simulink model "ASM_Traffic_V2X_Complete_Model_2"  (R2019a)
settings: Solver=ode1  StartTime=SIM.tstart.v  StopTime=Inf  FixedStep=SIM.StepSize.v  RelTol=1e-3
PostLoadFcn:
  | if any(exist('dsrtsu_mdlpostloadfcn', 'file') ~= 0), dsrtsu_mdlpostloadfcn('Execute', bdroot); end
  | try, asm_mdl_postloadfcn(bdroot, 'UpdateModel', 2200); catch, disp(lasterr); end,
undefined symbols (not defined in the file): _SensorPnts_1, _SensorPnts_13, _SensorPnts_17, _SensorPnts_21, _SensorPnts_25, _SensorPnts_29, _SensorPnts_33, _SensorPnts_37, _SensorPnts_41, _SensorPnts_45, _SensorPnts_49, _SensorPnts_5, _SensorPnts_53, _SensorPnts_57, _SensorPnts_9, _to_, CPT, G5A, ITS, MDL, rad, s_to_rpm, SIM
libraries: simulink x169, ASM_VehicleDynamics_lib x126, ASM_Traffic_lib x83, ASM_Utils_lib x49, mdbs x45, ASM_Environment_lib x17, dspindex x12, dsaV2xLibraryAux x10, dsmpblib x6, dsaV2xAsn1Library x4, dsaV2xLibrary x4, ASM_BrakeHydraulics_lib x4
(part 30 of 36)

== system ASM_Traffic_V2X_Complete_Model_2/MDLUserInterface/Environment/MDL_DISP/Traffic/Object_Sensor_2D/Object_Sensor_2D_VisualizationData/Sensor_5_Front_Right ==
  Sensor : Inport
  Angle_Hor_Rel[deg] : Gain
  Angle_ScopeZone_Horizontal[deg] : Gain
  Angle_z_Orientation_Sensor_CoorSys_V[deg] : Gain
  Bus Selector : BusSelector  OutputSignals=Parameters.Sensor_Enable[0Off|1On],Parameters.Sensor_Detection_Mode[1Ray|2Sector],Parameters.Length_ScopeZone[m],Parameters.Pos_Sensor_Apex_CoorSys_V[x;y;z][m],Parameters.Angle_z_Orientation_Sensor_CoorSys_V[deg],Parameters.Angle_ScopeZone_Horizontal[deg],Parameters.SensorIdx[],SensorOutput.Object_ID[],SensorOutput.Distance[m],SensorOutput.Angle_Hor_Rel[deg]
  Distance[m] : Gain
  Length_ScopeZone[m] : Gain
  Object_ID[] : Gain
  Pos_Sensor_Apex_CoorSys_V[x;y;z][m] : Gain
  SensorIdx[] : Gain
  Sensor_Detection_Mode[1Ray|2Sector] : Gain
  Sensor_Enable[0Off|1On] : Gain
  Terminator{,1..9} (10 alike) : Terminator
  wires:
  Bus Selector/3 -> Length_ScopeZone[m]/1  "<Length_ScopeZone[m]>"
  Length_ScopeZone[m]/1 -> Terminator9/1
  Bus Selector/10 -> Angle_Hor_Rel[deg]/1  "<Angle_Hor_Rel[deg]>"
  Bus Selector/9 -> Distance[m]/1  "<Distance[m]>"
  Bus Selector/8 -> Object_ID[]/1  "<Object_ID[]>"
  Bus Selector/7 -> SensorIdx[]/1  "<SensorIdx[]>"
  Bus Selector/6 -> Angle_ScopeZone_Horizontal[deg]/1  "<Angle_ScopeZone_Horizontal[deg]>"
  Bus Selector/5 -> Angle_z_Orientation_Sensor_CoorSys_V[deg]/1  "<Angle_z_Orientation_Sensor_CoorSys_V[deg]>"
  Bus Selector/4 -> Pos_Sensor_Apex_CoorSys_V[x;y;z][m]/1  "<Pos_Sensor_Apex_CoorSys_V[x;y;z][m]>"
  Angle_Hor_Rel[deg]/1 -> Terminator8/1
  Distance[m]/1 -> Terminator7/1
  Object_ID[]/1 -> Terminator6/1
  SensorIdx[]/1 -> Terminator5/1
  Angle_ScopeZone_Horizontal[deg]/1 -> Terminator4/1
  Angle_z_Orientation_Sensor_CoorSys_V[deg]/1 -> Terminator3/1
  Pos_Sensor_Apex_CoorSys_V[x;y;z][m]/1 -> Terminator2/1
  Bus Selector/2 -> Sensor_Detection_Mode[1Ray|2Sector]/1  "<Sensor_Detection_Mode[1Ray|2Sector]>"
  Sensor_Detection_Mode[1Ray|2Sector]/1 -> Terminator1/1
  Sensor_Enable[0Off|1On]/1 -> Terminator/1
  Bus Selector/1 -> Sensor_Enable[0Off|1On]/1  "<Sensor_Enable[0Off|1On]>"
  Sensor/1 -> Bus Selector/1

== system ASM_Traffic_V2X_Complete_Model_2/MDLUserInterface/Environment/MDL_DISP/Traffic/Object_Sensor_2D/Object_Sensor_2D_VisualizationData/Sensor_6_Right ==
  Sensor : Inport
  Angle_Hor_Rel[deg] : Gain
  Angle_ScopeZone_Horizontal[deg] : Gain
  Angle_z_Orientation_Sensor_CoorSys_V[deg] : Gain
  Bus Selector : BusSelector  OutputSignals=Parameters.Sensor_Enable[0Off|1On],Parameters.Sensor_Detection_Mode[1Ray|2Sector],Parameters.Length_ScopeZone[m],Parameters.Pos_Sensor_Apex_CoorSys_V[x;y;z][m],Parameters.Angle_z_Orientation_Sensor_CoorSys_V[deg],Parameters.Angle_ScopeZone_Horizontal[deg],Parameters.SensorIdx[],SensorOutput.Object_ID[],SensorOutput.Distance[m],SensorOutput.Angle_Hor_Rel[deg]
  Distance[m] : Gain
  Length_ScopeZone[m] : Gain
  Object_ID[] : Gain
  Pos_Sensor_Apex_CoorSys_V[x;y;z][m] : Gain
  SensorIdx[] : Gain
  Sensor_Detection_Mode[1Ray|2Sector] : Gain
  Sensor_Enable[0Off|1On] : Gain
  Terminator{,1..9} (10 alike) : Terminator
  wires:
  Sensor/1 -> Bus Selector/1
  Bus Selector/1 -> Sensor_Enable[0Off|1On]/1  "<Sensor_Enable[0Off|1On]>"
  Sensor_Enable[0Off|1On]/1 -> Terminator/1
  Sensor_Detection_Mode[1Ray|2Sector]/1 -> Terminator1/1
  Bus Selector/2 -> Sensor_Detection_Mode[1Ray|2Sector]/1  "<Sensor_Detection_Mode[1Ray|2Sector]>"
  Pos_Sensor_Apex_CoorSys_V[x;y;z][m]/1 -> Terminator2/1
  Angle_z_Orientation_Sensor_CoorSys_V[deg]/1 -> Terminator3/1
  Angle_ScopeZone_Horizontal[deg]/1 -> Terminator4/1
  SensorIdx[]/1 -> Terminator5/1
  Object_ID[]/1 -> Terminator6/1
  Distance[m]/1 -> Terminator7/1
  Angle_Hor_Rel[deg]/1 -> Terminator8/1
  Bus Selector/4 -> Pos_Sensor_Apex_CoorSys_V[x;y;z][m]/1  "<Pos_Sensor_Apex_CoorSys_V[x;y;z][m]>"
  Bus Selector/5 -> Angle_z_Orientation_Sensor_CoorSys_V[deg]/1  "<Angle_z_Orientation_Sensor_CoorSys_V[deg]>"
  Bus Selector/6 -> Angle_ScopeZone_Horizontal[deg]/1  "<Angle_ScopeZone_Horizontal[deg]>"
  Bus Selector/7 -> SensorIdx[]/1  "<SensorIdx[]>"
  Bus Selector/8 -> Object_ID[]/1  "<Object_ID[]>"
  Bus Selector/9 -> Distance[m]/1  "<Distance[m]>"
  Bus Selector/10 -> Angle_Hor_Rel[deg]/1  "<Angle_Hor_Rel[deg]>"
  Length_ScopeZone[m]/1 -> Terminator9/1
  Bus Selector/3 -> Length_ScopeZone[m]/1  "<Length_ScopeZone[m]>"

== system ASM_Traffic_V2X_Complete_Model_2/MDLUserInterface/Environment/MDL_DISP/Traffic/Object_Sensor_2D/Object_Sensor_2D_VisualizationData/Sensor_7_Rear_Right ==
  Sensor : Inport
  Angle_Hor_Rel[deg] : Gain
  Angle_ScopeZone_Horizontal[deg] : Gain
  Angle_z_Orientation_Sensor_CoorSys_V[deg] : Gain
  Bus Selector : BusSelector  OutputSignals=Parameters.Sensor_Enable[0Off|1On],Parameters.Sensor_Detection_Mode[1Ray|2Sector],Parameters.Length_ScopeZone[m],Parameters.Pos_Sensor_Apex_CoorSys_V[x;y;z][m],Parameters.Angle_z_Orientation_Sensor_CoorSys_V[deg],Parameters.Angle_ScopeZone_Horizontal[deg],Parameters.SensorIdx[],SensorOutput.Object_ID[],SensorOutput.Distance[m],SensorOutput.Angle_Hor_Rel[deg]
  Distance[m] : Gain
  Length_ScopeZone[m] : Gain
  Object_ID[] : Gain
  Pos_Sensor_Apex_CoorSys_V[x;y;z][m] : Gain
  SensorIdx[] : Gain
  Sensor_Detection_Mode[1Ray|2Sector] : Gain
  Sensor_Enable[0Off|1On] : Gain
  Terminator{,1..9} (10 alike) : Terminator
  wires:
  Bus Selector/3 -> Length_ScopeZone[m]/1  "<Length_ScopeZone[m]>"
  Length_ScopeZone[m]/1 -> Terminator9/1
  Bus Selector/10 -> Angle_Hor_Rel[deg]/1  "<Angle_Hor_Rel[deg]>"
  Bus Selector/9 -> Distance[m]/1  "<Distance[m]>"
  Bus Selector/8 -> Object_ID[]/1  "<Object_ID[]>"
  Bus Selector/7 -> SensorIdx[]/1  "<SensorIdx[]>"
  Bus Selector/6 -> Angle_ScopeZone_Horizontal[deg]/1  "<Angle_ScopeZone_Horizontal[deg]>"
  Bus Selector/5 -> Angle_z_Orientation_Sensor_CoorSys_V[deg]/1  "<Angle_z_Orientation_Sensor_CoorSys_V[deg]>"
  Bus Selector/4 -> Pos_Sensor_Apex_CoorSys_V[x;y;z][m]/1  "<Pos_Sensor_Apex_CoorSys_V[x;y;z][m]>"
  Angle_Hor_Rel[deg]/1 -> Terminator8/1
  Distance[m]/1 -> Terminator7/1
  Object_ID[]/1 -> Terminator6/1
  SensorIdx[]/1 -> Terminator5/1
  Angle_ScopeZone_Horizontal[deg]/1 -> Terminator4/1
  Angle_z_Orientation_Sensor_CoorSys_V[deg]/1 -> Terminator3/1
  Pos_Sensor_Apex_CoorSys_V[x;y;z][m]/1 -> Terminator2/1
  Bus Selector/2 -> Sensor_Detection_Mode[1Ray|2Sector]/1  "<Sensor_Detection_Mode[1Ray|2Sector]>"
  Sensor_Detection_Mode[1Ray|2Sector]/1 -> Terminator1/1
  Sensor_Enable[0Off|1On]/1 -> Terminator/1
  Bus Selector/1 -> Sensor_Enable[0Off|1On]/1  "<Sensor_Enable[0Off|1On]>"
  Sensor/1 -> Bus Selector/1

== system ASM_Traffic_V2X_Complete_Model_2/MDLUserInterface/Environment/MDL_DISP/Traffic/Object_Sensor_3D/IdxSelect_3DSensor/Angle_Hor_Object_1[deg] ==
  In1 : Inport
  Out1 : Outport
  wires:
  In1/1 -> Out1/1

== system ASM_Traffic_V2X_Complete_Model_2/MDLUserInterface/Environment/MDL_DISP/Traffic/Object_Sensor_3D/IdxSelect_3DSensor/Angle_Hor_Object_2[deg] ==
  In1 : Inport
  Out1 : Outport
  wires:
  In1/1 -> Out1/1

== system ASM_Traffic_V2X_Complete_Model_2/MDLUserInterface/Environment/MDL_DISP/Traffic/Object_Sensor_3D/IdxSelect_3DSensor/Angle_Hor_Object_3[deg] ==
  In1 : Inport
  Out1 : Outport
  wires:
  In1/1 -> Out1/1

== system ASM_Traffic_V2X_Complete_Model_2/MDLUserInterface/Environment/MDL_DISP/Traffic/Object_Sensor_3D/IdxSelect_3DSensor/Angle_Ver_Object_1[deg] ==
  In1 : Inport
  Out1 : Outport
  wires:
  In1/1 -> Out1/1

== system ASM_Traffic_V2X_Complete_Model_2/MDLUserInterface/Environment/MDL_DISP/Traffic/Object_Sensor_3D/IdxSelect_3DSensor/Angle_Ver_Object_2[deg] ==
  In1 : Inport
  Out1 : Outport
  wires:
  In1/1 -> Out1/1

== system ASM_Traffic_V2X_Complete_Model_2/MDLUserInterface/Environment/MDL_DISP/Traffic/Object_Sensor_3D/IdxSelect_3DSensor/Angle_Ver_Object_3[deg] ==
  In1 : Inport
  Out1 : Outport
  wires:
  In1/1 -> Out1/1

== system ASM_Traffic_V2X_Complete_Model_2/MDLUserInterface/Environment/MDL_DISP/Traffic/Object_Sensor_3D/IdxSelect_3DSensor/Dist_Object_1[m] ==
  In1 : Inport
  Out1 : Outport
  wires:
  In1/1 -> Out1/1

== system ASM_Traffic_V2X_Complete_Model_2/MDLUserInterface/Environment/MDL_DISP/Traffic/Object_Sensor_3D/IdxSelect_3DSensor/Dist_Object_2[m] ==
  In1 : Inport
  Out1 : Outport
  wires:
  In1/1 -> Out1/1

== system ASM_Traffic_V2X_Complete_Model_2/MDLUserInterface/Environment/MDL_DISP/Traffic/Object_Sensor_3D/IdxSelect_3DSensor/Dist_Object_3[m] ==
  In1 : Inport
  Out1 : Outport
  wires:
  In1/1 -> Out1/1

== system ASM_Traffic_V2X_Complete_Model_2/MDLUserInterface/Environment/MDL_DISP/Traffic/Object_Sensor_3D/IdxSelect_3DSensor/Flag_NearestPnt_Occluded1[-1|0|1] ==
  In1 : Inport
  Out1 : Outport
  wires:
  In1/1 -> Out1/1

== system ASM_Traffic_V2X_Complete_Model_2/MDLUserInterface/Environment/MDL_DISP/Traffic/Object_Sensor_3D/IdxSelect_3DSensor/Flag_NearestPnt_Occluded2[-1|0|1] ==
  In1 : Inport
  Out1 : Outport
  wires:
  In1/1 -> Out1/1

== system ASM_Traffic_V2X_Complete_Model_2/MDLUserInterface/Environment/MDL_DISP/Traffic/Object_Sensor_3D/IdxSelect_3DSensor/Flag_NearestPnt_Occluded3[-1|0|1] ==
  In1 : Inport
  Out1 : Outport
  wires:
  In1/1 -> Out1/1

== system ASM_Traffic_V2X_Complete_Model_2/MDLUserInterface/Environment/MDL_DISP/Traffic/Object_Sensor_3D/IdxSelect_3DSensor/Flag_Object_In_Scope_1[0Out|1In] ==
  In1 : Inport
  Out1 : Outport
  wires:
  In1/1 -> Out1/1

== system ASM_Traffic_V2X_Complete_Model_2/MDLUserInterface/Environment/MDL_DISP/Traffic/Object_Sensor_3D/IdxSelect_3DSensor/Flag_Object_In_Scope_2[0Out|1In] ==
  In1 : Inport
  Out1 : Outport
  wires:
  In1/1 -> Out1/1

== system ASM_Traffic_V2X_Complete_Model_2/MDLUserInterface/Environment/MDL_DISP/Traffic/Object_Sensor_3D/IdxSelect_3DSensor/Flag_Object_In_Scope_3[0Out|1In] ==
  In1 : Inport
  Out1 : Outport
  wires:
  In1/1 -> Out1/1

== system ASM_Traffic_V2X_Complete_Model_2/MDLUserInterface/Environment/MDL_DISP/Traffic/Object_Sensor_3D/IdxSelect_3DSensor/Flag_Sensor_Apex_In_Object_1[0Out|1In] ==
  In1 : Inport
  Out1 : Outport
  wires:
  In1/1 -> Out1/1

== system ASM_Traffic_V2X_Complete_Model_2/MDLUserInterface/Environment/MDL_DISP/Traffic/Object_Sensor_3D/IdxSelect_3DSensor/Flag_Sensor_Apex_In_Object_2[0Out|1In] ==
  In1 : Inport
  Out1 : Outport
  wires:
  In1/1 -> Out1/1

== system ASM_Traffic_V2X_Complete_Model_2/MDLUserInterface/Environment/MDL_DISP/Traffic/Object_Sensor_3D/IdxSelect_3DSensor/Flag_Sensor_Apex_In_Object_3[0Out|1In] ==
  In1 : Inport
  Out1 : Outport
  wires:
  In1/1 -> Out1/1

== system ASM_Traffic_V2X_Complete_Model_2/MDLUserInterface/Environment/MDL_DISP/Traffic/Object_Sensor_3D/IdxSelect_3DSensor/Object_ID_1[] ==
  In1 : Inport
  Out1 : Outport
  wires:
  In1/1 -> Out1/1

== system ASM_Traffic_V2X_Complete_Model_2/MDLUserInterface/Environment/MDL_DISP/Traffic/Object_Sensor_3D/IdxSelect_3DSensor/Object_ID_2[] ==
  In1 : Inport
  Out1 : Outport
  wires:
  In1/1 -> Out1/1

== system ASM_Traffic_V2X_Complete_Model_2/MDLUserInterface/Environment/MDL_DISP/Traffic/Object_Sensor_3D/IdxSelect_3DSensor/Object_ID_3[] ==
  In1 : Inport
  Out1 : Outport
  wires:
  In1/1 -> Out1/1

== system ASM_Traffic_V2X_Complete_Model_2/MDLUserInterface/Environment/MDL_DISP/Traffic/Object_Sensor_3D/IdxSelect_3DSensor/Object_Info_1[-1None|1Fellow|2Static] ==
  In1 : Inport
  Out1 : Outport
  wires:
  In1/1 -> Out1/1

== system ASM_Traffic_V2X_Complete_Model_2/MDLUserInterface/Environment/MDL_DISP/Traffic/Object_Sensor_3D/IdxSelect_3DSensor/Object_Info_2[-1None|1Fellow|2Static] ==
  In1 : Inport
  Out1 : Outport
  wires:
  In1/1 -> Out1/1

== system ASM_Traffic_V2X_Complete_Model_2/MDLUserInterface/Environment/MDL_DISP/Traffic/Object_Sensor_3D/IdxSelect_3DSensor/Object_Info_3[-1None|1Fellow|2Static] ==
  In1 : Inport
  Out1 : Outport
  wires:
  In1/1 -> Out1/1

== system ASM_Traffic_V2X_Complete_Model_2/MDLUserInterface/Environment/MDL_DISP/Traffic/Object_Sensor_3D/IdxSelect_3DSensor/Object_Type_1[] ==
  In1 : Inport
  Out1 : Outport
  wires:
  In1/1 -> Out1/1

== system ASM_Traffic_V2X_Complete_Model_2/MDLUserInterface/Environment/MDL_DISP/Traffic/Object_Sensor_3D/IdxSelect_3DSensor/Object_Type_2[] ==
  In1 : Inport
  Out1 : Outport
  wires:
  In1/1 -> Out1/1

== system ASM_Traffic_V2X_Complete_Model_2/MDLUserInterface/Environment/MDL_DISP/Traffic/Object_Sensor_3D/IdxSelect_3DSensor/Object_Type_3[] ==
  In1 : Inport
  Out1 : Outport
  wires:
  In1/1 -> Out1/1

== system ASM_Traffic_V2X_Complete_Model_2/MDLUserInterface/Environment/MDL_DISP/Traffic/Object_Sensor_3D/IdxSelect_3DSensor/Occlusion_Ratio_Object1[-1|0_1] ==
  In1 : Inport
  Out1 : Outport
  wires:
  In1/1 -> Out1/1

== system ASM_Traffic_V2X_Complete_Model_2/MDLUserInterface/Environment/MDL_DISP/Traffic/Object_Sensor_3D/IdxSelect_3DSensor/Occlusion_Ratio_Object2[-1|0_1] ==
  In1 : Inport
  Out1 : Outport
  wires:
  In1/1 -> Out1/1

== system ASM_Traffic_V2X_Complete_Model_2/MDLUserInterface/Environment/MDL_DISP/Traffic/Object_Sensor_3D/IdxSelect_3DSensor/Occlusion_Ratio_Object3[-1|0_1] ==
  In1 : Inport
  Out1 : Outport
  wires:
  In1/1 -> Out1/1

== system ASM_Traffic_V2X_Complete_Model_2/MDLUserInterface/Environment/MDL_DISP/Traffic/Object_Sensor_3D/IdxSelect_3DSensor/a_Rel_Object_1[m|s2] ==
  In1 : Inport
  Out1 : Outport
  wires:
  In1/1 -> Out1/1

== system ASM_Traffic_V2X_Complete_Model_2/MDLUserInterface/Environment/MDL_DISP/Traffic/Object_Sensor_3D/IdxSelect_3DSensor/a_Rel_Object_2[m|s2] ==
  In1 : Inport
  Out1 : Outport
  wires:
  In1/1 -> Out1/1

== system ASM_Traffic_V2X_Complete_Model_2/MDLUserInterface/Environment/MDL_DISP/Traffic/Object_Sensor_3D/IdxSelect_3DSensor/a_Rel_Object_3[m|s2] ==
  In1 : Inport
  Out1 : Outport
  wires:
  In1/1 -> Out1/1

== system ASM_Traffic_V2X_Complete_Model_2/MDLUserInterface/Environment/MDL_DISP/Traffic/Object_Sensor_3D/IdxSelect_3DSensor/v_Rel_Object_1[m|s] ==
  In1 : Inport
  Out1 : Outport
  wires:
  In1/1 -> Out1/1

== system ASM_Traffic_V2X_Complete_Model_2/MDLUserInterface/Environment/MDL_DISP/Traffic/Object_Sensor_3D/IdxSelect_3DSensor/v_Rel_Object_2[m|s] ==
  In1 : Inport
  Out1 : Outport
  wires:
  In1/1 -> Out1/1

== system ASM_Traffic_V2X_Complete_Model_2/MDLUserInterface/Environment/MDL_DISP/Traffic/Object_Sensor_3D/IdxSelect_3DSensor/v_Rel_Object_3[m|s] ==
  In1 : Inport
  Out1 : Outport
  wires:
  In1/1 -> Out1/1

== system ASM_Traffic_V2X_Complete_Model_2/MDLUserInterface/Environment/MDL_DISP/Traffic/Object_Sensor_3D/Object_Sensor_3D_VisualizationData/Sensor_1_Front_Long_CustomPoints ==
  Sensor : Inport
  Angle_Hor_Point[deg] : Gain
  Angle_Orientation_Sensor_CoorSys_V[x;y;z][deg] : Gain
  Angle_ScopeZone_Horizontal[deg] : Gain
  Bus Selector : BusSelector  OutputSignals=Parameter.Sensor_Enable[0Off|1On],Parameter.Geometry[],Parameter.Pos_Sensor_Apex_CoorSys_V[x;y;z][m],Parameter.Angle_Orientation_Sensor_CoorSys_V[x;y;z][deg],Parameter.Length_ScopeZone[m],Parameter.Length_ScopeZone_Head[m],Parameter.Angle_ScopeZone_Horizontal[deg],Parameter.Length_BlindZone[m],Parameter.SensorIdx[],CustomPoints.Object_ID[],CustomPoints.Dist_CoorSys_S[m],CustomPoints.Angle_Hor_CoorSys_S[deg]
  Dist_Point[m] : Gain
  Geometry[] : Gain
  Length_BlindZone[m] : Gain
  Length_ScopeZone[m] : Gain
  Length_ScopeZone_Head[m] : Gain
  Object_ID_Point[] : Gain
  Pos_Sensor_Apex_CoorSys_V[x;y;z][m] : Gain
  SensorIdx[] : Gain
  Sensor_Enable[0Off|1On] : Gain
  Terminator{9..20} (12 alike) : Terminator
  wires:
  Bus Selector/12 -> Angle_Hor_Point[deg]/1  "<Angle_Hor_CoorSys_S[deg]>"
  Bus Selector/10 -> Object_ID_Point[]/1  "<Object_ID[]>"
  Bus Selector/11 -> Dist_Point[m]/1  "<Dist_CoorSys_S[m]>"
  Bus Selector/9 -> SensorIdx[]/1  "<SensorIdx[]>"
  Bus Selector/8 -> Length_BlindZone[m]/1  "<Length_BlindZone[m]>"
  Bus Selector/7 -> Angle_ScopeZone_Horizontal[deg]/1  "<Angle_ScopeZone_Horizontal[deg]>"
  Bus Selector/6 -> Length_ScopeZone_Head[m]/1  "<Length_ScopeZone_Head[m]>"
  Bus Selector/5 -> Length_ScopeZone[m]/1  "<Length_ScopeZone[m]>"
  Bus Selector/4 -> Angle_Orientation_Sensor_CoorSys_V[x;y;z][deg]/1  "<Angle_Orientation_Sensor_CoorSys_V[x;y;z][deg]>"
  Bus Selector/3 -> Pos_Sensor_Apex_CoorSys_V[x;y;z][m]/1  "<Pos_Sensor_Apex_CoorSys_V[x;y;z][m]>"
  Bus Selector/2 -> Geometry[]/1  "<Geometry[]>"
  Bus Selector/1 -> Sensor_Enable[0Off|1On]/1  "<Sensor_Enable[0Off|1On]>"
  Object_ID_Point[]/1 -> Terminator13/1
  Geometry[]/1 -> Terminator11/1
  Pos_Sensor_Apex_CoorSys_V[x;y;z][m]/1 -> Terminator20/1
  Length_ScopeZone_Head[m]/1 -> Terminator16/1
  SensorIdx[]/1 -> Terminator14/1
  Angle_Hor_Point[deg]/1 -> Terminator19/1
  Angle_Orientation_Sensor_CoorSys_V[x;y;z][deg]/1 -> Terminator18/1
  Dist_Point[m]/1 -> Terminator9/1
  Length_ScopeZone[m]/1 -> Terminator17/1
  Sensor_Enable[0Off|1On]/1 -> Terminator10/1
  Angle_ScopeZone_Horizontal[deg]/1 -> Terminator15/1
  Length_BlindZone[m]/1 -> Terminator12/1
  Sensor/1 -> Bus Selector/1

== system ASM_Traffic_V2X_Complete_Model_2/MDLUserInterface/Environment/MDL_DISP/Traffic/Object_Sensor_3D/Object_Sensor_3D_VisualizationData/Sensor_1_Front_Long_NearestPoints ==
  Sensor : Inport
  Angle_Hor_Point[deg] : Gain
  Angle_Orientation_Sensor_CoorSys_V[x;y;z][deg] : Gain
  Angle_ScopeZone_Horizontal[deg] : Gain
  Bus Selector : BusSelector  OutputSignals=Parameter.Sensor_Enable[0Off|1On],Parameter.Geometry[],Parameter.Pos_Sensor_Apex_CoorSys_V[x;y;z][m],Parameter.Angle_Orientation_Sensor_CoorSys_V[x;y;z][deg],Parameter.Length_ScopeZone[m],Parameter.Length_ScopeZone_Head[m],Parameter.Angle_ScopeZone_Horizontal[deg],Parameter.Length_BlindZone[m],Parameter.SensorIdx[],SensorOutput.Object_ID[],SensorOutput.Dist_Object[m],SensorOutput.Angle_Hor_Object[deg]
  Dist_Point[m] : Gain
  Geometry[] : Gain
  Length_BlindZone[m] : Gain
  Length_ScopeZone[m] : Gain
  Length_ScopeZone_Head[m] : Gain
  Object_ID_Point[] : Gain
  Pos_Sensor_Apex_CoorSys_V[x;y;z][m] : Gain
  SensorIdx[] : Gain
  Sensor_Enable[0Off|1On] : Gain
  Terminator{9..20} (12 alike) : Terminator
  wires:
  Bus Selector/12 -> Angle_Hor_Point[deg]/1  "<Angle_Hor_Object[deg]>"
  Bus Selector/10 -> Object_ID_Point[]/1  "<Object_ID[]>"
  Bus Selector/11 -> Dist_Point[m]/1  "<Dist_Object[m]>"
  Bus Selector/9 -> SensorIdx[]/1  "<SensorIdx[]>"
  Bus Selector/8 -> Length_BlindZone[m]/1  "<Length_BlindZone[m]>"
  Bus Selector/7 -> Angle_ScopeZone_Horizontal[deg]/1  "<Angle_ScopeZone_Horizontal[deg]>"
  Bus Selector/6 -> Length_ScopeZone_Head[m]/1  "<Length_ScopeZone_Head[m]>"
  Bus Selector/5 -> Length_ScopeZone[m]/1  "<Length_ScopeZone[m]>"
  Bus Selector/4 -> Angle_Orientation_Sensor_CoorSys_V[x;y;z][deg]/1  "<Angle_Orientation_Sensor_CoorSys_V[x;y;z][deg]>"
  Bus Selector/3 -> Pos_Sensor_Apex_CoorSys_V[x;y;z][m]/1  "<Pos_Sensor_Apex_CoorSys_V[x;y;z][m]>"
  Bus Selector/2 -> Geometry[]/1  "<Geometry[]>"
  Bus Selector/1 -> Sensor_Enable[0Off|1On]/1  "<Sensor_Enable[0Off|1On]>"
  Object_ID_Point[]/1 -> Terminator13/1
  Geometry[]/1 -> Terminator11/1
  Pos_Sensor_Apex_CoorSys_V[x;y;z][m]/1 -> Terminator20/1
  Length_ScopeZone_Head[m]/1 -> Terminator16/1
  SensorIdx[]/1 -> Terminator14/1
  Angle_Hor_Point[deg]/1 -> Terminator19/1
  Angle_Orientation_Sensor_CoorSys_V[x;y;z][deg]/1 -> Terminator18/1
  Dist_Point[m]/1 -> Terminator9/1
  Length_ScopeZone[m]/1 -> Terminator17/1
  Sensor_Enable[0Off|1On]/1 -> Terminator10/1
  Angle_ScopeZone_Horizontal[deg]/1 -> Terminator15/1
  Length_BlindZone[m]/1 -> Terminator12/1
  Sensor/1 -> Bus Selector/1

== system ASM_Traffic_V2X_Complete_Model_2/MDLUserInterface/Environment/MDL_DISP/Traffic/Object_Sensor_3D/Object_Sensor_3D_VisualizationData/Sensor_1_Front_Long_RadarReflectionPoints ==
  Sensor : Inport
  Angle_Hor_Point[deg] : Gain
  Angle_Orientation_Sensor_CoorSys_V[x;y;z][deg] : Gain
  Angle_ScopeZone_Horizontal[deg] : Gain
  Bus Selector : BusSelector  OutputSignals=Parameter.Sensor_Enable[0Off|1On],Parameter.Geometry[],Parameter.Pos_Sensor_Apex_CoorSys_V[x;y;z][m],Parameter.Angle_Orientation_Sensor_CoorSys_V[x;y;z][deg],Parameter.Length_ScopeZone[m],Parameter.Length_ScopeZone_Head[m],Parameter.Angle_ScopeZone_Horizontal[deg],Parameter.Length_BlindZone[m],Parameter.SensorIdx[],RadarEffects.Object_ID[],RadarEffects.Dist_CoorSys_S[m],RadarEffects.Angle_Hor_CoorSys_S[deg]
  Dist_Point[m] : Gain
  Geometry[] : Gain
  Length_BlindZone[m] : Gain
  Length_ScopeZone[m] : Gain
  Length_ScopeZone_Head[m] : Gain
  Object_ID_Point[] : Gain
  Pos_Sensor_Apex_CoorSys_V[x;y;z][m] : Gain
  SensorIdx[] : Gain
  Sensor_Enable[0Off|1On] : Gain
  Terminator{9..20} (12 alike) : Terminator
  wires:
  Sensor/1 -> Bus Selector/1
  Length_BlindZone[m]/1 -> Terminator12/1
  Angle_ScopeZone_Horizontal[deg]/1 -> Terminator15/1
  Sensor_Enable[0Off|1On]/1 -> Terminator10/1
  Length_ScopeZone[m]/1 -> Terminator17/1
  Dist_Point[m]/1 -> Terminator9/1
  Angle_Orientation_Sensor_CoorSys_V[x;y;z][deg]/1 -> Terminator18/1
  Angle_Hor_Point[deg]/1 -> Terminator19/1
  SensorIdx[]/1 -> Terminator14/1
  Length_ScopeZone_Head[m]/1 -> Terminator16/1
  Pos_Sensor_Apex_CoorSys_V[x;y;z][m]/1 -> Terminator20/1
  Geometry[]/1 -> Terminator11/1
  Object_ID_Point[]/1 -> Terminator13/1
  Bus Selector/1 -> Sensor_Enable[0Off|1On]/1  "<Sensor_Enable[0Off|1On]>"
  Bus Selector/2 -> Geometry[]/1  "<Geometry[]>"
  Bus Selector/3 -> Pos_Sensor_Apex_CoorSys_V[x;y;z][m]/1  "<Pos_Sensor_Apex_CoorSys_V[x;y;z][m]>"
  Bus Selector/4 -> Angle_Orientation_Sensor_CoorSys_V[x;y;z][deg]/1  "<Angle_Orientation_Sensor_CoorSys_V[x;y;z][deg]>"
  Bus Selector/5 -> Length_ScopeZone[m]/1  "<Length_ScopeZone[m]>"
  Bus Selector/6 -> Length_ScopeZone_Head[m]/1  "<Length_ScopeZone_Head[m]>"
  Bus Selector/7 -> Angle_ScopeZone_Horizontal[deg]/1  "<Angle_ScopeZone_Horizontal[deg]>"
  Bus Selector/8 -> Length_BlindZone[m]/1  "<Length_BlindZone[m]>"
  Bus Selector/9 -> SensorIdx[]/1  "<SensorIdx[]>"
  Bus Selector/11 -> Dist_Point[m]/1  "<Dist_CoorSys_S[m]>"
  Bus Selector/10 -> Object_ID_Point[]/1  "<Object_ID[]>"
  Bus Selector/12 -> Angle_Hor_Point[deg]/1  "<Angle_Hor_CoorSys_S[deg]>"

== system ASM_Traffic_V2X_Complete_Model_2/MDLUserInterface/Environment/MDL_DISP/Traffic/Object_Sensor_3D/Object_Sensor_3D_VisualizationData/Sensor_2_Front_Mid_CustomPoints ==
  Sensor : Inport
  Angle_Hor_Point[deg] : Gain
  Angle_Orientation_Sensor_CoorSys_V[x;y;z][deg] : Gain
  Angle_ScopeZone_Horizontal[deg] : Gain
  Bus Selector : BusSelector  OutputSignals=Parameter.Sensor_Enable[0Off|1On],Parameter.Geometry[],Parameter.Pos_Sensor_Apex_CoorSys_V[x;y;z][m],Parameter.Angle_Orientation_Sensor_CoorSys_V[x;y;z][deg],Parameter.Length_ScopeZone[m],Parameter.Length_ScopeZone_Head[m],Parameter.Angle_ScopeZone_Horizontal[deg],Parameter.Length_BlindZone[m],Parameter.SensorIdx[],CustomPoints.Object_ID[],CustomPoints.Dist_CoorSys_S[m],CustomPoints.Angle_Hor_CoorSys_S[deg]
  Dist_Point[m] : Gain
  Geometry[] : Gain
  Length_BlindZone[m] : Gain
  Length_ScopeZone[m] : Gain
  Length_ScopeZone_Head[m] : Gain
  Object_ID_Point[] : Gain
  Pos_Sensor_Apex_CoorSys_V[x;y;z][m] : Gain
  SensorIdx[] : Gain
  Sensor_Enable[0Off|1On] : Gain
  Terminator{9..20} (12 alike) : Terminator
  wires:
  Sensor/1 -> Bus Selector/1
  Length_BlindZone[m]/1 -> Terminator12/1
  Angle_ScopeZone_Horizontal[deg]/1 -> Terminator15/1
  Sensor_Enable[0Off|1On]/1 -> Terminator10/1
  Length_ScopeZone[m]/1 -> Terminator17/1
  Dist_Point[m]/1 -> Terminator9/1
  Angle_Orientation_Sensor_CoorSys_V[x;y;z][deg]/1 -> Terminator18/1
  Angle_Hor_Point[deg]/1 -> Terminator19/1
  SensorIdx[]/1 -> Terminator14/1
  Length_ScopeZone_Head[m]/1 -> Terminator16/1
  Pos_Sensor_Apex_CoorSys_V[x;y;z][m]/1 -> Terminator20/1
  Geometry[]/1 -> Terminator11/1
  Object_ID_Point[]/1 -> Terminator13/1
  Bus Selector/1 -> Sensor_Enable[0Off|1On]/1  "<Sensor_Enable[0Off|1On]>"
  Bus Selector/2 -> Geometry[]/1  "<Geometry[]>"
  Bus Selector/3 -> Pos_Sensor_Apex_CoorSys_V[x;y;z][m]/1  "<Pos_Sensor_Apex_CoorSys_V[x;y;z][m]>"
  Bus Selector/4 -> Angle_Orientation_Sensor_CoorSys_V[x;y;z][deg]/1  "<Angle_Orientation_Sensor_CoorSys_V[x;y;z][deg]>"
  Bus Selector/5 -> Length_ScopeZone[m]/1  "<Length_ScopeZone[m]>"
  Bus Selector/6 -> Length_ScopeZone_Head[m]/1  "<Length_ScopeZone_Head[m]>"
  Bus Selector/7 -> Angle_ScopeZone_Horizontal[deg]/1  "<Angle_ScopeZone_Horizontal[deg]>"
  Bus Selector/8 -> Length_BlindZone[m]/1  "<Length_BlindZone[m]>"
  Bus Selector/9 -> SensorIdx[]/1  "<SensorIdx[]>"
  Bus Selector/11 -> Dist_Point[m]/1  "<Dist_CoorSys_S[m]>"
  Bus Selector/10 -> Object_ID_Point[]/1  "<Object_ID[]>"
  Bus Selector/12 -> Angle_Hor_Point[deg]/1  "<Angle_Hor_CoorSys_S[deg]>"

== system ASM_Traffic_V2X_Complete_Model_2/MDLUserInterface/Environment/MDL_DISP/Traffic/Object_Sensor_3D/Object_Sensor_3D_VisualizationData/Sensor_2_Front_Mid_NearestPoints ==
  Sensor : Inport
  Angle_Hor_Point[deg] : Gain
  Angle_Orientation_Sensor_CoorSys_V[x;y;z][deg] : Gain
  Angle_ScopeZone_Horizontal[deg] : Gain
  Bus Selector : BusSelector  OutputSignals=Parameter.Sensor_Enable[0Off|1On],Parameter.Geometry[],Parameter.Pos_Sensor_Apex_CoorSys_V[x;y;z][m],Parameter.Angle_Orientation_Sensor_CoorSys_V[x;y;z][deg],Parameter.Length_ScopeZone[m],Parameter.Length_ScopeZone_Head[m],Parameter.Angle_ScopeZone_Horizontal[deg],Parameter.Length_BlindZone[m],Parameter.SensorIdx[],SensorOutput.Object_ID[],SensorOutput.Dist_Object[m],SensorOutput.Angle_Hor_Object[deg]
  Dist_Point[m] : Gain
  Geometry[] : Gain
  Length_BlindZone[m] : Gain
  Length_ScopeZone[m] : Gain
  Length_ScopeZone_Head[m] : Gain
  Object_ID_Point[] : Gain
  Pos_Sensor_Apex_CoorSys_V[x;y;z][m] : Gain
  SensorIdx[] : Gain
  Sensor_Enable[0Off|1On] : Gain
  Terminator{9..20} (12 alike) : Terminator
  wires:
  Sensor/1 -> Bus Selector/1
  Length_BlindZone[m]/1 -> Terminator12/1
  Angle_ScopeZone_Horizontal[deg]/1 -> Terminator15/1
  Sensor_Enable[0Off|1On]/1 -> Terminator10/1
  Length_ScopeZone[m]/1 -> Terminator17/1
  Dist_Point[m]/1 -> Terminator9/1
  Angle_Orientation_Sensor_CoorSys_V[x;y;z][deg]/1 -> Terminator18/1
  Angle_Hor_Point[deg]/1 -> Terminator19/1
  SensorIdx[]/1 -> Terminator14/1
  Length_ScopeZone_Head[m]/1 -> Terminator16/1
  Pos_Sensor_Apex_CoorSys_V[x;y;z][m]/1 -> Terminator20/1
  Geometry[]/1 -> Terminator11/1
  Object_ID_Point[]/1 -> Terminator13/1
  Bus Selector/1 -> Sensor_Enable[0Off|1On]/1  "<Sensor_Enable[0Off|1On]>"
  Bus Selector/2 -> Geometry[]/1  "<Geometry[]>"
  Bus Selector/3 -> Pos_Sensor_Apex_CoorSys_V[x;y;z][m]/1  "<Pos_Sensor_Apex_CoorSys_V[x;y;z][m]>"
  Bus Selector/4 -> Angle_Orientation_Sensor_CoorSys_V[x;y;z][deg]/1  "<Angle_Orientation_Sensor_CoorSys_V[x;y;z][deg]>"
  Bus Selector/5 -> Length_ScopeZone[m]/1  "<Length_ScopeZone[m]>"
  Bus Selector/6 -> Length_ScopeZone_Head[m]/1  "<Length_ScopeZone_Head[m]>"
  Bus Selector/7 -> Angle_ScopeZone_Horizontal[deg]/1  "<Angle_ScopeZone_Horizontal[deg]>"
  Bus Selector/8 -> Length_BlindZone[m]/1  "<Length_BlindZone[m]>"
  Bus Selector/9 -> SensorIdx[]/1  "<SensorIdx[]>"
  Bus Selector/11 -> Dist_Point[m]/1  "<Dist_Object[m]>"
  Bus Selector/10 -> Object_ID_Point[]/1  "<Object_ID[]>"
  Bus Selector/12 -> Angle_Hor_Point[deg]/1  "<Angle_Hor_Object[deg]>"

== system ASM_Traffic_V2X_Complete_Model_2/MDLUserInterface/Environment/MDL_DISP/Traffic/Object_Sensor_3D/Object_Sensor_3D_VisualizationData/Sensor_2_Front_Mid_RadarReflectionPoints ==
  Sensor : Inport
  Angle_Hor_Point[deg] : Gain
  Angle_Orientation_Sensor_CoorSys_V[x;y;z][deg] : Gain
  Angle_ScopeZone_Horizontal[deg] : Gain
  Bus Selector : BusSelector  OutputSignals=Parameter.Sensor_Enable[0Off|1On],Parameter.Geometry[],Parameter.Pos_Sensor_Apex_CoorSys_V[x;y;z][m],Parameter.Angle_Orientation_Sensor_CoorSys_V[x;y;z][deg],Parameter.Length_ScopeZone[m],Parameter.Length_ScopeZone_Head[m],Parameter.Angle_ScopeZone_Horizontal[deg],Parameter.Length_BlindZone[m],Parameter.SensorIdx[],RadarEffects.Object_ID[],RadarEffects.Dist_CoorSys_S[m],RadarEffects.Angle_Hor_CoorSys_S[deg]
  Dist_Point[m] : Gain
  Geometry[] : Gain
  Length_BlindZone[m] : Gain
  Length_ScopeZone[m] : Gain
  Length_ScopeZone_Head[m] : Gain
  Object_ID_Point[] : Gain
  Pos_Sensor_Apex_CoorSys_V[x;y;z][m] : Gain
  SensorIdx[] : Gain
  Sensor_Enable[0Off|1On] : Gain
  Terminator{9..20} (12 alike) : Terminator
  wires:
  Bus Selector/12 -> Angle_Hor_Point[deg]/1  "<Angle_Hor_CoorSys_S[deg]>"
  Bus Selector/10 -> Object_ID_Point[]/1  "<Object_ID[]>"
  Bus Selector/11 -> Dist_Point[m]/1  "<Dist_CoorSys_S[m]>"
  Bus Selector/9 -> SensorIdx[]/1  "<SensorIdx[]>"
  Bus Selector/8 -> Length_BlindZone[m]/1  "<Length_BlindZone[m]>"
  Bus Selector/7 -> Angle_ScopeZone_Horizontal[deg]/1  "<Angle_ScopeZone_Horizontal[deg]>"
  Bus Selector/6 -> Length_ScopeZone_Head[m]/1  "<Length_ScopeZone_Head[m]>"
  Bus Selector/5 -> Length_ScopeZone[m]/1  "<Length_ScopeZone[m]>"
  Bus Selector/4 -> Angle_Orientation_Sensor_CoorSys_V[x;y;z][deg]/1  "<Angle_Orientation_Sensor_CoorSys_V[x;y;z][deg]>"
  Bus Selector/3 -> Pos_Sensor_Apex_CoorSys_V[x;y;z][m]/1  "<Pos_Sensor_Apex_CoorSys_V[x;y;z][m]>"
  Bus Selector/2 -> Geometry[]/1  "<Geometry[]>"
  Bus Selector/1 -> Sensor_Enable[0Off|1On]/1  "<Sensor_Enable[0Off|1On]>"
  Object_ID_Point[]/1 -> Terminator13/1
  Geometry[]/1 -> Terminator11/1
  Pos_Sensor_Apex_CoorSys_V[x;y;z][m]/1 -> Terminator20/1
  Length_ScopeZone_Head[m]/1 -> Terminator16/1
  SensorIdx[]/1 -> Terminator14/1
  Angle_Hor_Point[deg]/1 -> Terminator19/1
  Angle_Orientation_Sensor_CoorSys_V[x;y;z][deg]/1 -> Terminator18/1
  Dist_Point[m]/1 -> Terminator9/1
  Length_ScopeZone[m]/1 -> Terminator17/1
  Sensor_Enable[0Off|1On]/1 -> Terminator10/1
  Angle_ScopeZone_Horizontal[deg]/1 -> Terminator15/1
  Length_BlindZone[m]/1 -> Terminator12/1
  Sensor/1 -> Bus Selector/1

== system ASM_Traffic_V2X_Complete_Model_2/MDLUserInterface/Environment/MDL_DISP/Traffic/Object_Sensor_3D/Object_Sensor_3D_VisualizationData/Sensor_3_Rear_CustomPoints ==
  Sensor : Inport
  Angle_Hor_Point[deg] : Gain
  Angle_Orientation_Sensor_CoorSys_V[x;y;z][deg] : Gain
  Angle_ScopeZone_Horizontal[deg] : Gain
  Bus Selector : BusSelector  OutputSignals=Parameter.Sensor_Enable[0Off|1On],Parameter.Geometry[],Parameter.Pos_Sensor_Apex_CoorSys_V[x;y;z][m],Parameter.Angle_Orientation_Sensor_CoorSys_V[x;y;z][deg],Parameter.Length_ScopeZone[m],Parameter.Length_ScopeZone_Head[m],Parameter.Angle_ScopeZone_Horizontal[deg],Parameter.Length_BlindZone[m],Parameter.SensorIdx[],CustomPoints.Object_ID[],CustomPoints.Dist_CoorSys_S[m],CustomPoints.Angle_Hor_CoorSys_S[deg]
  Dist_Point[m] : Gain
  Geometry[] : Gain
  Length_BlindZone[m] : Gain
  Length_ScopeZone[m] : Gain
  Length_ScopeZone_Head[m] : Gain
  Object_ID_Point[] : Gain
  Pos_Sensor_Apex_CoorSys_V[x;y;z][m] : Gain
  SensorIdx[] : Gain
  Sensor_Enable[0Off|1On] : Gain
  Terminator{9..20} (12 alike) : Terminator
  wires:
  Bus Selector/12 -> Angle_Hor_Point[deg]/1  "<Angle_Hor_CoorSys_S[deg]>"
  Bus Selector/10 -> Object_ID_Point[]/1  "<Object_ID[]>"
  Bus Selector/11 -> Dist_Point[m]/1  "<Dist_CoorSys_S[m]>"
  Bus Selector/9 -> SensorIdx[]/1  "<SensorIdx[]>"
  Bus Selector/8 -> Length_BlindZone[m]/1  "<Length_BlindZone[m]>"
  Bus Selector/7 -> Angle_ScopeZone_Horizontal[deg]/1  "<Angle_ScopeZone_Horizontal[deg]>"
  Bus Selector/6 -> Length_ScopeZone_Head[m]/1  "<Length_ScopeZone_Head[m]>"
  Bus Selector/5 -> Length_ScopeZone[m]/1  "<Length_ScopeZone[m]>"
  Bus Selector/4 -> Angle_Orientation_Sensor_CoorSys_V[x;y;z][deg]/1  "<Angle_Orientation_Sensor_CoorSys_V[x;y;z][deg]>"
  Bus Selector/3 -> Pos_Sensor_Apex_CoorSys_V[x;y;z][m]/1  "<Pos_Sensor_Apex_CoorSys_V[x;y;z][m]>"
  Bus Selector/2 -> Geometry[]/1  "<Geometry[]>"
  Bus Selector/1 -> Sensor_Enable[0Off|1On]/1  "<Sensor_Enable[0Off|1On]>"
  Object_ID_Point[]/1 -> Terminator13/1
  Geometry[]/1 -> Terminator11/1
  Pos_Sensor_Apex_CoorSys_V[x;y;z][m]/1 -> Terminator20/1
  Length_ScopeZone_Head[m]/1 -> Terminator16/1
  SensorIdx[]/1 -> Terminator14/1
  Angle_Hor_Point[deg]/1 -> Terminator19/1
  Angle_Orientation_Sensor_CoorSys_V[x;y;z][deg]/1 -> Terminator18/1
  Dist_Point[m]/1 -> Terminator9/1
  Length_ScopeZone[m]/1 -> Terminator17/1
  Sensor_Enable[0Off|1On]/1 -> Terminator10/1
  Angle_ScopeZone_Horizontal[deg]/1 -> Terminator15/1
  Length_BlindZone[m]/1 -> Terminator12/1
  Sensor/1 -> Bus Selector/1

== system ASM_Traffic_V2X_Complete_Model_2/MDLUserInterface/Environment/MDL_DISP/Traffic/Object_Sensor_3D/Object_Sensor_3D_VisualizationData/Sensor_3_Rear_NearestPoints ==
  Sensor : Inport
  Angle_Hor_Point[deg] : Gain
  Angle_Orientation_Sensor_CoorSys_V[x;y;z][deg] : Gain
  Angle_ScopeZone_Horizontal[deg] : Gain
  Bus Selector : BusSelector  OutputSignals=Parameter.Sensor_Enable[0Off|1On],Parameter.Geometry[],Parameter.Pos_Sensor_Apex_CoorSys_V[x;y;z][m],Parameter.Angle_Orientation_Sensor_CoorSys_V[x;y;z][deg],Parameter.Length_ScopeZone[m],Parameter.Length_ScopeZone_Head[m],Parameter.Angle_ScopeZone_Horizontal[deg],Parameter.Length_BlindZone[m],Parameter.SensorIdx[],SensorOutput.Object_ID[],SensorOutput.Dist_Object[m],SensorOutput.Angle_Hor_Object[deg]
  Dist_Point[m] : Gain
  Geometry[] : Gain
  Length_BlindZone[m] : Gain
  Length_ScopeZone[m] : Gain
  Length_ScopeZone_Head[m] : Gain
  Object_ID_Point[] : Gain
  Pos_Sensor_Apex_CoorSys_V[x;y;z][m] : Gain
  SensorIdx[] : Gain
  Sensor_Enable[0Off|1On] : Gain
  Terminator{9..20} (12 alike) : Terminator
  wires:
  Bus Selector/12 -> Angle_Hor_Point[deg]/1  "<Angle_Hor_Object[deg]>"
  Bus Selector/10 -> Object_ID_Point[]/1  "<Object_ID[]>"
  Bus Selector/11 -> Dist_Point[m]/1  "<Dist_Object[m]>"
  Bus Selector/9 -> SensorIdx[]/1  "<SensorIdx[]>"
  Bus Selector/8 -> Length_BlindZone[m]/1  "<Length_BlindZone[m]>"
  Bus Selector/7 -> Angle_ScopeZone_Horizontal[deg]/1  "<Angle_ScopeZone_Horizontal[deg]>"
  Bus Selector/6 -> Length_ScopeZone_Head[m]/1  "<Length_ScopeZone_Head[m]>"
  Bus Selector/5 -> Length_ScopeZone[m]/1  "<Length_ScopeZone[m]>"
  Bus Selector/4 -> Angle_Orientation_Sensor_CoorSys_V[x;y;z][deg]/1  "<Angle_Orientation_Sensor_CoorSys_V[x;y;z][deg]>"
  Bus Selector/3 -> Pos_Sensor_Apex_CoorSys_V[x;y;z][m]/1  "<Pos_Sensor_Apex_CoorSys_V[x;y;z][m]>"
  Bus Selector/2 -> Geometry[]/1  "<Geometry[]>"
  Bus Selector/1 -> Sensor_Enable[0Off|1On]/1  "<Sensor_Enable[0Off|1On]>"
  Object_ID_Point[]/1 -> Terminator13/1
  Geometry[]/1 -> Terminator11/1
  Pos_Sensor_Apex_CoorSys_V[x;y;z][m]/1 -> Terminator20/1
  Length_ScopeZone_Head[m]/1 -> Terminator16/1
  SensorIdx[]/1 -> Terminator14/1
  Angle_Hor_Point[deg]/1 -> Terminator19/1
  Angle_Orientation_Sensor_CoorSys_V[x;y;z][deg]/1 -> Terminator18/1
  Dist_Point[m]/1 -> Terminator9/1
  Length_ScopeZone[m]/1 -> Terminator17/1
  Sensor_Enable[0Off|1On]/1 -> Terminator10/1
  Angle_ScopeZone_Horizontal[deg]/1 -> Terminator15/1
  Length_BlindZone[m]/1 -> Terminator12/1
  Sensor/1 -> Bus Selector/1

== system ASM_Traffic_V2X_Complete_Model_2/MDLUserInterface/Environment/MDL_DISP/Traffic/Object_Sensor_3D/Object_Sensor_3D_VisualizationData/Sensor_3_Rear_RadarReflectionPoints ==
  Sensor : Inport
  Angle_Hor_Point[deg] : Gain
  Angle_Orientation_Sensor_CoorSys_V[x;y;z][deg] : Gain
  Angle_ScopeZone_Horizontal[deg] : Gain
  Bus Selector : BusSelector  OutputSignals=Parameter.Sensor_Enable[0Off|1On],Parameter.Geometry[],Parameter.Pos_Sensor_Apex_CoorSys_V[x;y;z][m],Parameter.Angle_Orientation_Sensor_CoorSys_V[x;y;z][deg],Parameter.Length_ScopeZone[m],Parameter.Length_ScopeZone_Head[m],Parameter.Angle_ScopeZone_Horizontal[deg],Parameter.Length_BlindZone[m],Parameter.SensorIdx[],RadarEffects.Object_ID[],RadarEffects.Dist_CoorSys_S[m],RadarEffects.Angle_Hor_CoorSys_S[deg]
  Dist_Point[m] : Gain
  Geometry[] : Gain
  Length_BlindZone[m] : Gain
  Length_ScopeZone[m] : Gain
  Length_ScopeZone_Head[m] : Gain
  Object_ID_Point[] : Gain
  Pos_Sensor_Apex_CoorSys_V[x;y;z][m] : Gain
  SensorIdx[] : Gain
  Sensor_Enable[0Off|1On] : Gain
  Terminator{9..20} (12 alike) : Terminator
  wires:
  Sensor/1 -> Bus Selector/1
  Length_BlindZone[m]/1 -> Terminator12/1
  Angle_ScopeZone_Horizontal[deg]/1 -> Terminator15/1
  Sensor_Enable[0Off|1On]/1 -> Terminator10/1
  Length_ScopeZone[m]/1 -> Terminator17/1
  Dist_Point[m]/1 -> Terminator9/1
  Angle_Orientation_Sensor_CoorSys_V[x;y;z][deg]/1 -> Terminator18/1
  Angle_Hor_Point[deg]/1 -> Terminator19/1
  SensorIdx[]/1 -> Terminator14/1
  Length_ScopeZone_Head[m]/1 -> Terminator16/1
  Pos_Sensor_Apex_CoorSys_V[x;y;z][m]/1 -> Terminator20/1
  Geometry[]/1 -> Terminator11/1
  Object_ID_Point[]/1 -> Terminator13/1
  Bus Selector/1 -> Sensor_Enable[0Off|1On]/1  "<Sensor_Enable[0Off|1On]>"
  Bus Selector/2 -> Geometry[]/1  "<Geometry[]>"
  Bus Selector/3 -> Pos_Sensor_Apex_CoorSys_V[x;y;z][m]/1  "<Pos_Sensor_Apex_CoorSys_V[x;y;z][m]>"
  Bus Selector/4 -> Angle_Orientation_Sensor_CoorSys_V[x;y;z][deg]/1  "<Angle_Orientation_Sensor_CoorSys_V[x;y;z][deg]>"
  Bus Selector/5 -> Length_ScopeZone[m]/1  "<Length_ScopeZone[m]>"
  Bus Selector/6 -> Length_ScopeZone_Head[m]/1  "<Length_ScopeZone_Head[m]>"
  Bus Selector/7 -> Angle_ScopeZone_Horizontal[deg]/1  "<Angle_ScopeZone_Horizontal[deg]>"
  Bus Selector/8 -> Length_BlindZone[m]/1  "<Length_BlindZone[m]>"
  Bus Selector/9 -> SensorIdx[]/1  "<SensorIdx[]>"
  Bus Selector/11 -> Dist_Point[m]/1  "<Dist_CoorSys_S[m]>"
  Bus Selector/10 -> Object_ID_Point[]/1  "<Object_ID[]>"
  Bus Selector/12 -> Angle_Hor_Point[deg]/1  "<Angle_Hor_CoorSys_S[deg]>"

== system ASM_Traffic_V2X_Complete_Model_2/MDLUserInterface/Environment/MDL_DISP/Traffic/Traffic_Sign_Sensor/GetTrfSgnDataByIndex_1/SwitchObjectData ==
  TrafficBus : Inport
  Switch : Inport  Port=2
  Bus Selector2 : BusSelector  OutputSignals=Sensors.TrafficSign_Sensor_Dyn.Sensor_Front_1.SensorOutput[].TrafficObject_Type[]
  Bus Selector3 : BusSelector  OutputSignals=Sensors.TrafficSign_Sensor_Dyn.Sensor_Front_1.SensorOutput[].TrafficObject_ID[]
  Bus Selector4 : BusSelector  OutputSignals=Sensors.TrafficSign_Sensor_Dyn.Sensor_Front_1.SensorOutput[].Parent_Object_ID[]
  Bus Selector44 : BusSelector  OutputSignals=Sensors.TrafficSign_Sensor_Dyn.Sensor_Front_1.SensorOutput[].Traffic_Sign_Valid[0|1]
  Selector{,1..3} (4 alike) : Selector  InputPortWidth=MDL.Traffic.Sensors.TrafficSignSensorDyn_Calculation.Const_Sensor_Output_Dimension.v  IndexOptions=Index vector (port)  Indices=[1 3]  OutputSizes=1
  Traffic_Sign_Valid[0|1] : Outport
  TrafficObject_ID[] : Outport  Port=2
  TrafficObject_Type[] : Outport  Port=3
  Parent_Object_ID[] : Outport  Port=4
  wires:
  Bus Selector2/1 -> Selector2/1  "<TrafficObject_Type[]>"
  TrafficBus/1 -> Bus Selector4/1, Bus Selector2/1, Bus Selector3/1, Bus Selector44/1
  Bus Selector3/1 -> Selector1/1  "<TrafficObject_ID[]>"
  Selector1/1 -> TrafficObject_ID[]/1
  Bus Selector44/1 -> Selector/1  "<Traffic_Sign_Valid[0|1]>"
  Selector/1 -> Traffic_Sign_Valid[0|1]/1
  Switch/1 -> Selector3/2, Selector2/2, Selector1/2, Selector/2
  Selector2/1 -> TrafficObject_Type[]/1
  Bus Selector4/1 -> Selector3/1  "<Parent_Object_ID[]>"
  Selector3/1 -> Parent_Object_ID[]/1

== system ASM_Traffic_V2X_Complete_Model_2/MDLUserInterface/Environment/MDL_DISP/Traffic/Traffic_Sign_Sensor/GetTrfSgnDataByIndex_1/SwitchObjectPosition ==
  TrafficBus : Inport
  Switch : Inport  Port=2
  Bus Selector1 : BusSelector  OutputSignals=Sensors.TrafficSign_Sensor_Dyn.Sensor_Front_1.SensorOutput[].Pos_CoorSys_S[x;y;z][m]
  Bus Selector2 : BusSelector  OutputSignals=Sensors.TrafficSign_Sensor_Dyn.Sensor_Front_1.SensorOutput[].Angle_Hor_Rel[deg]
  Bus Selector3 : BusSelector  OutputSignals=Sensors.TrafficSign_Sensor_Dyn.Sensor_Front_1.SensorOutput[].Angle_CoorSys_E[x;y;z][deg]
  Bus Selector4 : BusSelector  OutputSignals=Sensors.TrafficSign_Sensor_Dyn.Sensor_Front_1.SensorOutput[].Angle_Ver_Rel[deg]
  Bus Selector44 : BusSelector  OutputSignals=Sensors.TrafficSign_Sensor_Dyn.Sensor_Front_1.SensorOutput[].Pos_CoorSys_E[x;y;z][m]
  Bus Selector5 : BusSelector  OutputSignals=Sensors.TrafficSign_Sensor_Dyn.Sensor_Front_1.SensorOutput[].Distance[m]
  Idx_comp : Subsystem
  Idx_comp1 : Subsystem
  Idx_comp2 : Subsystem
  Mux : Mux  Inputs=3
  Mux1 : Mux  Inputs=3
  Mux2 : Mux  Inputs=3
  Selector{1..9} (9 alike) : Selector  InputPortWidth=MDL.Traffic.Sensors.TrafficSignSensorDyn_Calculation.Const_Sensor_Output_Dimension.v*3  IndexOptions=Index vector (port)  Indices=[1 3]  OutputSizes=1
  Selector10 : Selector  InputPortWidth=MDL.Traffic.Sensors.TrafficSignSensorDyn_Calculation.Const_Sensor_Output_Dimension.v  IndexOptions=Index vector (port)  Indices=[1 3]  OutputSizes=1
  Selector11 : Selector  InputPortWidth=MDL.Traffic.Sensors.TrafficSignSensorDyn_Calculation.Const_Sensor_Output_Dimension.v  IndexOptions=Index vector (port)  Indices=[1 3]  OutputSizes=1
  Selector12 : Selector  InputPortWidth=MDL.Traffic.Sensors.TrafficSignSensorDyn_Calculation.Const_Sensor_Output_Dimension.v  IndexOptions=Index vector (port)  Indices=[1 3]  OutputSizes=1
  Pos_CoorSys_E[x;y;z][m] : Outport
  Angle_CoorSys_E[x;y;z][deg] : Outport  Port=2
  Pos_CoorSys_S[x;y;z][m] : Outport  Port=3
  Angle_Hor_Rel[deg] : Outport  Port=4
  Angle_Ver_Rel[deg] : Outport  Port=5
  Distance[m] : Outport  Port=6
  wires:
  Switch/1 -> Selector12/2, Selector11/2, Selector10/2, Idx_comp2/1(Idx), Idx_comp1/1(Idx), Idx_comp/1(Idx)
  Bus Selector44/1 -> Selector6/1, Selector5/1, Selector4/1  "<Pos_CoorSys_E[x;y;z][m]>"
  Bus Selector3/1 -> Selector3/1, Selector2/1, Selector1/1  "<Angle_CoorSys_E[x;y;z][deg]>"
  TrafficBus/1 -> Bus Selector44/1, Bus Selector5/1, Bus Selector4/1, Bus Selector2/1, Bus Selector1/1, Bus Selector3/1
  Idx_comp/1(Idx_comp_x) -> Selector4/2
  Idx_comp/2(Idx_comp_y) -> Selector5/2
  Idx_comp/3(Idx_comp_z) -> Selector6/2
  Selector4/1 -> Mux/1
  Selector5/1 -> Mux/2
  Selector6/1 -> Mux/3
  Mux/1 -> Pos_CoorSys_E[x;y;z][m]/1
  Idx_comp1/1(Idx_comp_x) -> Selector1/2
  Idx_comp1/2(Idx_comp_y) -> Selector2/2
  Idx_comp1/3(Idx_comp_z) -> Selector3/2
  Selector1/1 -> Mux1/1
  Selector2/1 -> Mux1/2
  Selector3/1 -> Mux1/3
  Mux1/1 -> Angle_CoorSys_E[x;y;z][deg]/1
  Bus Selector1/1 -> Selector9/1, Selector8/1, Selector7/1  "<Pos_CoorSys_S[x;y;z][m]>"
  Selector7/1 -> Mux2/1
  Selector8/1 -> Mux2/2
  Selector9/1 -> Mux2/3
  Idx_comp2/1(Idx_comp_x) -> Selector7/2
  Idx_comp2/2(Idx_comp_y) -> Selector8/2
  Idx_comp2/3(Idx_comp_z) -> Selector9/2
  Mux2/1 -> Pos_CoorSys_S[x;y;z][m]/1
  Bus Selector2/1 -> Selector10/1  "<Angle_Hor_Rel[deg]>"
  Bus Selector4/1 -> Selector11/1  "<Angle_Ver_Rel[deg]>"
  Bus Selector5/1 -> Selector12/1  "<Distance[m]>"
  Selector10/1 -> Angle_Hor_Rel[deg]/1
  Selector11/1 -> Angle_Ver_Rel[deg]/1
  Selector12/1 -> Distance[m]/1

== system ASM_Traffic_V2X_Complete_Model_2/MDLUserInterface/Environment/MDL_DISP/Traffic/Traffic_Sign_Sensor/GetTrfSgnDataByIndex_1/SwitchSignProperties ==
  TrafficBus : Inport
  Switch : Inport  Port=2
  Bus Selector1 : BusSelector  OutputSignals=Sensors.TrafficSign_Sensor_Dyn.Sensor_Front_1.SensorOutput[].Traffic_Sign_Visibility[0_100]
  Bus Selector2 : BusSelector  OutputSignals=Sensors.TrafficSign_Sensor_Dyn.Sensor_Front_1.SensorOutput[].Traffic_Sign_Value[]
  Bus Selector3 : BusSelector  OutputSignals=Sensors.TrafficSign_Sensor_Dyn.Sensor_Front_1.SensorOutput[].Traffic_Sign_Subtype[]
  Bus Selector4 : BusSelector  OutputSignals=Sensors.TrafficSign_Sensor_Dyn.Sensor_Front_1.SensorOutput[].Traffic_Sign_Country[]
  Bus Selector44 : BusSelector  OutputSignals=Sensors.TrafficSign_Sensor_Dyn.Sensor_Front_1.SensorOutput[].Traffic_Sign_Type[]
  Bus Selector5 : BusSelector  OutputSignals=Sensors.TrafficSign_Sensor_Dyn.Sensor_Front_1.SensorOutput[].Traffic_Sign_Lanes[]
  Bus Selector6 : BusSelector  OutputSignals=Sensors.TrafficSign_Sensor_Dyn.Sensor_Front_1.SensorOutput[].Object_State[]
  Bus Selector7 : BusSelector  OutputSignals=Sensors.TrafficSign_Sensor_Dyn.Sensor_Front_1.SensorOutput[].Object_Stream_ID[]
  Idx_comp : Subsystem
  Mux2 : Mux  Inputs=5
  Selector{,1..3,6,10..11} (7 alike) : Selector  InputPortWidth=MDL.Traffic.Sensors.TrafficSignSensorDyn_Calculation.Const_Sensor_Output_Dimension.v  IndexOptions=Index vector (port)  Indices=[1 3]  OutputSizes=1
  Selector{4..5,7..9} (5 alike) : Selector  InputPortWidth=MDL.Traffic.Sensors.TrafficSignSensorDyn_Calculation.Const_Sensor_Output_Dimension.v*5  IndexOptions=Index vector (port)  Indices=[1 3]  OutputSizes=1
  Traffic_Sign_Type[] : Outport
  Traffic_Sign_Subtype[] : Outport  Port=2
  Traffic_Sign_Value[] : Outport  Port=3
  Traffic_Sign_Country[] : Outport  Port=4
  Traffic_Sign_Visibility[0_100] : Outport  Port=5
  Object_State[] : Outport  Port=6
  Object_Stream_ID[] : Outport  Port=7
  Traffic_Sign_Lanes[] : Outport  Port=8
  wires:
  Selector3/1 -> Traffic_Sign_Country[]/1
  Bus Selector4/1 -> Selector3/1  "<Traffic_Sign_Country[]>"
  Selector2/1 -> Traffic_Sign_Value[]/1
  Switch/1 -> Selector/2, Selector1/2, Selector2/2, Selector6/2, Selector11/2, Idx_comp/1(Idx), Selector10/2, Selector3/2
  Selector/1 -> Traffic_Sign_Type[]/1
  Bus Selector44/1 -> Selector/1  "<Traffic_Sign_Type[]>"
  Selector1/1 -> Traffic_Sign_Subtype[]/1
  Bus Selector3/1 -> Selector1/1  "<Traffic_Sign_Subtype[]>"
  TrafficBus/1 -> Bus Selector44/1, Bus Selector3/1, Bus Selector2/1, Bus Selector6/1, Bus Selector5/1, Bus Selector7/1, Bus Selector1/1, Bus Selector4/1
  Bus Selector2/1 -> Selector2/1  "<Traffic_Sign_Value[]>"
  Bus Selector1/1 -> Selector6/1  "<Traffic_Sign_Visibility[0_100]>"
  Bus Selector5/1 -> Selector4/1, Selector5/1, Selector9/1, Selector8/1, Selector7/1  "<Traffic_Sign_Lanes[]>"
  Selector7/1 -> Mux2/1
  Selector8/1 -> Mux2/2
  Selector9/1 -> Mux2/3
  Idx_comp/1(Idx_comp_1) -> Selector7/2
  Idx_comp/2(Idx_comp_2) -> Selector8/2
  Idx_comp/3(Idx_comp_3) -> Selector9/2
  Mux2/1 -> Traffic_Sign_Lanes[]/1
  Selector5/1 -> Mux2/5
  Idx_comp/5(Idx_comp_5) -> Selector5/2
  Idx_comp/4(Idx_comp_4) -> Selector4/2
  Selector4/1 -> Mux2/4
  Selector6/1 -> Traffic_Sign_Visibility[0_100]/1
  Selector10/1 -> Object_State[]/1
  Bus Selector6/1 -> Selector10/1  "<Object_State[]>"
  Selector11/1 -> Object_Stream_ID[]/1
  Bus Selector7/1 -> Selector11/1  "<Object_Stream_ID[]>"

== system ASM_Traffic_V2X_Complete_Model_2/MDLUserInterface/MotionDeskInterface/MOTION_DESK_INTERFACE/Traffic_Animation/Sensors_Animation/Sensor_Points/Line_Sensor_Junction_Border_Points ==
  ModelSignals : Inport
  Bus Selector : BusSelector  OutputSignals=Pos_x_Junction_Border_Animation_CoorSys_E,Pos_y_Junction_Border_Animation_CoorSys_E,Pos_z_Junction_Border_Animation_CoorSys_E
  CC : Concatenate  NumInputs=4  Mode=Multidimensional array
  Reshape1 : Reshape  OutputDimensionality=Row vector (2-D)
  Reshape2 : Reshape  OutputDimensionality=Row vector (2-D)
  Reshape3 : Reshape  OutputDimensionality=Row vector (2-D)
  zero : Constant  Value=zeros(1,60)  VectorParams1D=off
  AnimationSignals : Outport
  wires:
  ModelSignals/1 -> Bus Selector/1
  CC/1 -> AnimationSignals/1
  Bus Selector/1 -> Reshape1/1  "<Pos_x_Junction_Border_Animation_CoorSys_E>"
  Bus Selector/2 -> Reshape2/1  "<Pos_y_Junction_Border_Animation_CoorSys_E>"
  Bus Selector/3 -> Reshape3/1  "<Pos_z_Junction_Border_Animation_CoorSys_E>"
  Reshape1/1 -> CC/1
  Reshape2/1 -> CC/2
  Reshape3/1 -> CC/3
  zero/1 -> CC/4

== system ASM_Traffic_V2X_Complete_Model_2/MDLUserInterface/MotionDeskInterface/MOTION_DESK_INTERFACE/Traffic_Animation/Sensors_Animation/Sensor_Points/Line_Sensor_Junction_Shape_ContObj_Points ==
  ModelSignals : Inport
  Bus Selector : BusSelector  OutputSignals=Pos_x_Junction_Shape_ContObj_Animation_CoorSys_E,Pos_y_Junction_Shape_ContObj_Animation_CoorSys_E,Pos_z_Junction_Shape_ContObj_Animation_CoorSys_E
  CC : Concatenate  NumInputs=4  Mode=Multidimensional array
  Reshape1 : Reshape  OutputDimensionality=Row vector (2-D)
  Reshape2 : Reshape  OutputDimensionality=Row vector (2-D)
  Reshape3 : Reshape  OutputDimensionality=Row vector (2-D)
  zero : Constant  Value=zeros(1,60)  VectorParams1D=off
  AnimationSignals : Outport
  wires:
  ModelSignals/1 -> Bus Selector/1
  CC/1 -> AnimationSignals/1
  Bus Selector/1 -> Reshape1/1  "<Pos_x_Junction_Shape_ContObj_Animation_CoorSys_E>"
  Bus Selector/2 -> Reshape2/1  "<Pos_y_Junction_Shape_ContObj_Animation_CoorSys_E>"
  Bus Selector/3 -> Reshape3/1  "<Pos_z_Junction_Shape_ContObj_Animation_CoorSys_E>"
  Reshape1/1 -> CC/1
  Reshape2/1 -> CC/2
  Reshape3/1 -> CC/3
  zero/1 -> CC/4
